simulink model "tcpipSf17a"  (R2017a)
settings: Solver=VariableStepAuto  StartTime=0.0  StopTime=10.0  RelTol=1e-3
settings Model: Creator=aoyuchen  LastModifiedBy=diliou

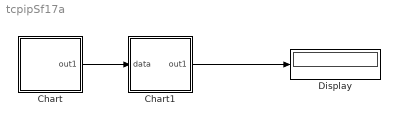
== system tcpipSf17a ==
  Chart : Stateflow chart  TreatAsAtomicUnit=on
  Chart1 : Stateflow chart  TreatAsAtomicUnit=on
  Display : Display
  wires:
  Chart1/1(out1) -> Display/1
  Chart/1(out1) -> Chart1/1(data)

== stateflow chart tcpipSf17a/Chart1 ==
  state A
    en,du:
    out1 = tcpGet;
  (default) -> A
  data: y function_output; out1 output double =1; data input
  function y = tcpGet:
    | function y = tcpGet
    | persistent obj
    | y = 1;
    | coder.extrinsic('evalin');
    | coder.extrinsic('get');
    | if isempty(obj)
    |     obj = evalin('base','objWs');
    | end
    | bytesAvail=get(obj,'InputBufferSize');
    | y = bytesAvail;

== stateflow chart tcpipSf17a/Chart ==
  state A
    en,du:
    tcpInit;
    out1 = 0;
  (default) -> A
  data: out1 output
  function tcpInit:
    | function tcpInit
    | coder.extrinsic('tcpip');
    | coder.extrinsic('assignin');
    | persistent obj
    | if isempty(obj)
    |     obj=tcpip('rhost','InputBufferSize',780);
    |     assignin('base','objWs',obj);
    | end
